simulink model "FLIGHT_hexacopter"  (R2024a)
settings: Solver=FixedStepDiscrete  StartTime=0.0  StopTime=inf  FixedStep=SampleTime_SAS  RelTol=1e-3  EnableMultiTasking=on
InitFcn:
  | Init_FLIGHT_Hexacopter
values from neighbouring files (symbols this model uses):
  d2r = pi/180    (= 0.0174532925199)    [Init_FLIGHT_Hexacopter.m]
  Kdpr = 0.004    [Init_FLIGHT_Hexacopter_fromNCMS.m]
  Kdrr = 0.004    [Init_FLIGHT_Hexacopter_fromNCMS.m]
  Kdvz = 0.0254    [Init_FLIGHT_Hexacopter_fromNCMS.m]
  Kdyr = 0.0298    [Init_FLIGHT_Hexacopter_fromNCMS.m]
  Kipr = 0.0    (= 0)    [Init_FLIGHT_Hexacopter_fromNCMS.m]
  Kirr = 0.0    (= 0)    [Init_FLIGHT_Hexacopter_fromNCMS.m]
  Kivz = 0.6304    [Init_FLIGHT_Hexacopter_fromNCMS.m]
  Kiyr = 0.0    (= 0)    [Init_FLIGHT_Hexacopter_fromNCMS.m]
  Kpp = 3.3894    [Init_FLIGHT_Hexacopter_fromNCMS.m]
  Kppr = 0.1    [Init_FLIGHT_Hexacopter_fromNCMS.m]
  Kpr = 3.3894    [Init_FLIGHT_Hexacopter_fromNCMS.m]
  Kprr = 0.1    [Init_FLIGHT_Hexacopter_fromNCMS.m]
  Kpvz = 0.3191    [Init_FLIGHT_Hexacopter_fromNCMS.m]
  Kpyr = 0.3744    [Init_FLIGHT_Hexacopter_fromNCMS.m]
  MAX_CONTROL_ANGLE_PITCH = 30*pi/180    (= 0.523598775598)    [Init_FLIGHT_Hexacopter.m]    (also in Init_FLIGHT_Hexacopter_fromNCMS.m = 0.349065850399)
  MAX_CONTROL_ANGLE_RATE_PITCH = 360*pi/180    (= 6.28318530718)    [Init_FLIGHT_Hexacopter.m]    (also in Init_FLIGHT_Hexacopter_fromNCMS.m)
  MAX_CONTROL_ANGLE_RATE_ROLL = 360*pi/180    (= 6.28318530718)    [Init_FLIGHT_Hexacopter.m]    (also in Init_FLIGHT_Hexacopter_fromNCMS.m)
  MAX_CONTROL_ANGLE_RATE_Y = 120*pi/180    (= 2.09439510239)    [Init_FLIGHT_Hexacopter.m]    (also in Init_FLIGHT_Hexacopter_fromNCMS.m)
  MAX_CONTROL_ANGLE_ROLL = 30*pi/180    (= 0.523598775598)    [Init_FLIGHT_Hexacopter.m]    (also in Init_FLIGHT_Hexacopter_fromNCMS.m = 0.349065850399)
  MAX_CONTROL_VELOCITY_XY = 1.5    [Init_FLIGHT_Hexacopter.m]    (also in Init_FLIGHT_Hexacopter_fromNCMS.m)
  MAX_CONTROL_VELOCITY_Z = 1    [Init_FLIGHT_Hexacopter.m]    (also in Init_FLIGHT_Hexacopter_fromNCMS.m)
  Npr = 50    [Init_FLIGHT_Hexacopter_fromNCMS.m]
  Nrr = 50    [Init_FLIGHT_Hexacopter_fromNCMS.m]
  Nvz = Npr    (= 50)    [Init_FLIGHT_Hexacopter_fromNCMS.m]
  Nyr = 50    [Init_FLIGHT_Hexacopter_fromNCMS.m]
  SampleTime = 1/200    (= 0.005)    [Init_FLIGHT_Hexacopter.m]    (also in Init_FLIGHT_Hexacopter_fromNCMS.m = 0.01)
  SampleTime_SAS = 1/1000    (= 0.001)    [Init_FLIGHT_Hexacopter.m]
undefined symbols (not defined in the file or in its folder): arguments, event_sequence, id, log_levels, MPC_Z_D, MPC_Z_I, MPC_Z_P, noutputs, output, pitch, pitch_body, q_d, roll, roll_body, thrust_body, timestamp, vx, vy, vz, x, y, yaw, yaw_sp_move_rate, z
libraries: px4lib x35, px4uORBlib x12, px4Utilslib x11, slpidlib x10, simulink x3, simulink_extras x2, px4Sensorslib x2, sharedtransform x1
(part 2 of 3)

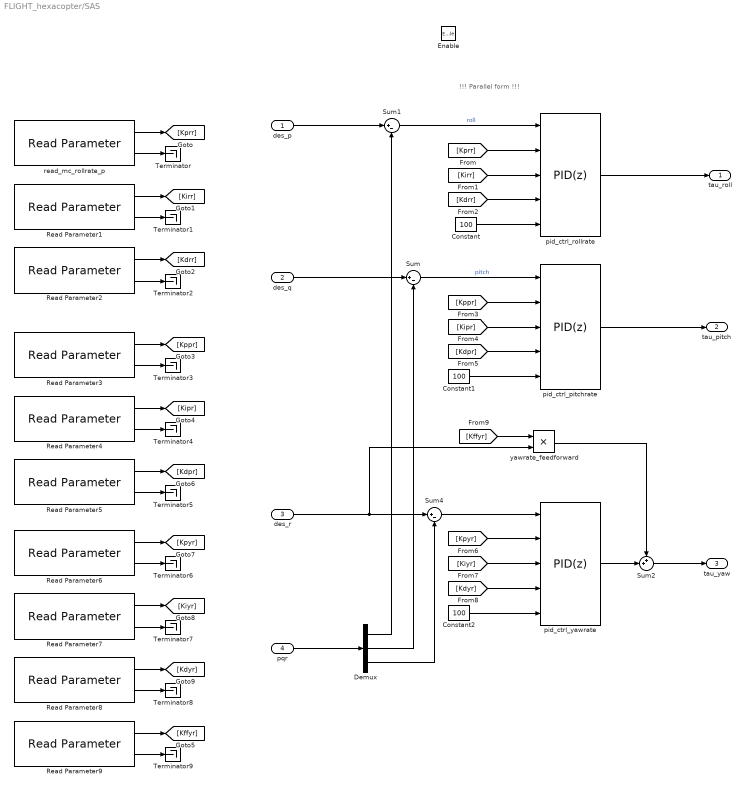
== system FLIGHT_hexacopter/SAS ==
  note: !!! Parallel form !!!
  des_p : Inport
  des_q : Inport  Port=2
  des_r : Inport  Port=3
  pqr : Inport  Port=4
  Enable : EnablePort
  Constant : Constant  Value=100  OutDataTypeStr=single  SampleTime=SampleTime_SAS
  Constant1 : Constant  Value=100  OutDataTypeStr=single  SampleTime=SampleTime_SAS
  Constant2 : Constant  Value=100  OutDataTypeStr=single  SampleTime=SampleTime_SAS
  Demux : Demux  Outputs=3
  Read Parameter1 : px4lib/Read Parameter  ParameterName=MC_ROLLRATE_I  DataType=FLOAT  SampleTime=SampleTime_SAS
      settings: SourceProductName=UAV Toolbox Support Package for PX4 Autopilots
  Read Parameter2 : px4lib/Read Parameter  ParameterName=MC_ROLLRATE_D  DataType=FLOAT  SampleTime=SampleTime_SAS
      settings: SourceProductName=UAV Toolbox Support Package for PX4 Autopilots
  Read Parameter3 : px4lib/Read Parameter  ParameterName=MC_PITCHRATE_P  DataType=FLOAT  SampleTime=SampleTime_SAS
      settings: SourceProductName=UAV Toolbox Support Package for PX4 Autopilots
  Read Parameter4 : px4lib/Read Parameter  ParameterName=MC_PITCHRATE_I  DataType=FLOAT  SampleTime=SampleTime_SAS
      settings: SourceProductName=UAV Toolbox Support Package for PX4 Autopilots
  Read Parameter5 : px4lib/Read Parameter  ParameterName=MC_PITCHRATE_D  DataType=FLOAT  SampleTime=SampleTime_SAS
      settings: SourceProductName=UAV Toolbox Support Package for PX4 Autopilots
  Read Parameter6 : px4lib/Read Parameter  ParameterName=MC_YAWRATE_P  DataType=FLOAT  SampleTime=SampleTime_SAS
      settings: SourceProductName=UAV Toolbox Support Package for PX4 Autopilots
  Read Parameter7 : px4lib/Read Parameter  ParameterName=MC_YAWRATE_I  DataType=FLOAT  SampleTime=SampleTime_SAS
      settings: SourceProductName=UAV Toolbox Support Package for PX4 Autopilots
  Read Parameter8 : px4lib/Read Parameter  ParameterName=MC_YAWRATE_D  DataType=FLOAT  SampleTime=SampleTime_SAS
      settings: SourceProductName=UAV Toolbox Support Package for PX4 Autopilots
  Read Parameter9 : px4lib/Read Parameter  ParameterName=MC_YAWRATE_FF  DataType=FLOAT  SampleTime=SampleTime_SAS
      settings: SourceProductName=UAV Toolbox Support Package for PX4 Autopilots
  Sum : Sum  Inputs=|+-
  Sum1 : Sum  Inputs=|+-
  Sum2 : Sum  Inputs=++|
  Sum4 : Sum  Inputs=|+-
  Terminator{,1..9} (10 alike) : Terminator
  pid_ctrl_pitchrate : slpidlib/PID Controller  Controller=PID  Form=Parallel  TimeDomain=Discrete-time  UseExternalTs=off  SampleTime=SampleTime_SAS  IntegratorMethod=Forward Euler  FilterMethod=Forward Euler  ControllerParametersSource=external  P=Kppr  I=Kipr  UseKiTs=off  D=Kdpr  UseExternalDerivativeSource=off  N=Npr  UseFilter=on  TunerSelectOption=Transfer Function Based (PID Tuner App)  InitialConditionSource=internal  InitialConditionForIntegrator=0  InitialConditionForFilter=0  DifferentiatorICPrevScaledInput=0  ExternalReset=none  TrackingMode=off  Kt=1  LimitOutput=off  SatLimitsSource=internal  UpperSaturationLimit=0.2  LowerSaturationLimit=-0.2  LinearizeAsGain=on  AntiWindupMode=clamping  Kb=1  LimitIntegrator=off  UpperIntegratorSaturationLimit=inf  LowerIntegratorSaturationLimit=-inf  POutMin=[]  POutMax=[]  IOutMin=[]  IOutMax=[]  DOutMin=[]  DOutMax=[]  NOutMin=[]  NOutMax=[]  SumOutMin=[]  SumOutMax=[]  SaturationOutDataTypeStr=single  SaturationOutMin=[]  SaturationOutMax=[]  PParamMin=[]  PParamMax=[]  IParamMin=[]  IParamMax=[]  DParamMin=[]  DParamMax=[]  NParamMin=[]  NParamMax=[]  KbParamMin=[]  KbParamMax=[]  KtParamMin=[]  KtParamMax=[]  KbOutMin=[]  KbOutMax=[]  KtOutMin=[]  KtOutMax=[]  IntegratorOutMin=[]  IntegratorOutMax=[]  FilterOutMin=[]  FilterOutMax=[]  SumI1OutMin=[]  SumI1OutMax=[]  SumI2OutMin=[]  SumI2OutMax=[]  SumI3OutMin=[]  SumI3OutMax=[]  SumI4OutMin=[]  SumI4OutMax=[]  SumDOutMin=[]  SumDOutMax=[]  DifferentiatorOutMin=[]  DifferentiatorOutMax=[]  FilterDiffOutCoefMin=[]  FilterDiffOutCoefMax=[]  ReciprocalOutMin=[]  ReciprocalOutMax=[]  SumDenOutMin=[]  SumDenOutMax=[]  SumNumOutMin=[]  SumNumOutMax=[]  DivideOutMin=[]  DivideOutMax=[]  UdiffTsProdOutMin=[]  UdiffTsProdOutMax=[]  NTsProdOutMin=[]  NTsProdOutMax=[]  UintegralTsProdOutMin=[]  UintegralTsProdOutMax=[]  UngainTsProdOutMin=[]  UngainTsProdOutMax=[]  ClampingZeroOutDataTypeStr=Inherit: Inherit via back propagation  ClampingZeroOutMin=[]  ClampingZeroOutMax=[]  FilterDenConstantOutDataTypeStr=Inherit: Inherit via back propagation  FilterDenConstantOutMin=[]  FilterDenConstantOutMax=[]  PCopyOutDataTypeStr=Inherit: Inherit via back propagation  PCopyOutMin=[]  PCopyOutMax=[]  NCopyOutDataTypeStr=Inherit: Inherit via back propagation  NCopyOutMin=[]  NCopyOutMax=[]  IntegratorContinuousStateAttributes=''  IntegratorStateMustResolveToSignalObject=off  IntegratorRTWStateStorageClass=Auto  FilterContinuousStateAttributes=''  FilterStateMustResolveToSignalObject=off  FilterRTWStateStorageClass=Auto  ParallelPVariant=ExternalParameters  IdealPVariant=Disabled  IVariant=ExternalParameters  DVariant=ExternalParameters  IntegratorVariant=Discrete  SatVariant=Disabled  AWVariant=Passthrough  PCopyVariant=Disabled  TRVariant=Disabled  FdbkBlocksVariant=Forward  IdealPFdbkVariant=Disabled  SatFdbkVariant=Disabled  DerivativeFilterVariant=ForwardEulerFilter  NVariant=ExternalParameters  NCopyVariant=Disabled  FilterICVariant=InternalICsFilter  IntegratorICVariant=InternalICs  ExternalResetVariant=Disabled  TRSumVariant=Passthrough  SumFdbkVariant=Disabled  SumVariant=Sum_PID  TsampFilterVariant=InternalTs  TsampNgainVariant=Passthrough  TsampIntegralVariant=Disabled_SignalSpec  ExternalSaturationOutDataTypeStr=single  DerivativeSourceVariant=ErrorSignal
  pid_ctrl_rollrate : slpidlib/PID Controller  Controller=PID  Form=Parallel  TimeDomain=Discrete-time  UseExternalTs=off  SampleTime=SampleTime_SAS  IntegratorMethod=Forward Euler  FilterMethod=Forward Euler  ControllerParametersSource=external  P=Kprr  I=Kirr  UseKiTs=off  D=Kdrr  UseExternalDerivativeSource=off  N=Nrr  UseFilter=on  TunerSelectOption=Transfer Function Based (PID Tuner App)  InitialConditionSource=internal  InitialConditionForIntegrator=0  InitialConditionForFilter=0  DifferentiatorICPrevScaledInput=0  ExternalReset=none  TrackingMode=off  Kt=1  LimitOutput=off  SatLimitsSource=internal  UpperSaturationLimit=0.2  LowerSaturationLimit=-0.2  LinearizeAsGain=on  AntiWindupMode=clamping  Kb=1  LimitIntegrator=off  UpperIntegratorSaturationLimit=inf  LowerIntegratorSaturationLimit=-inf  POutMin=[]  POutMax=[]  IOutMin=[]  IOutMax=[]  DOutMin=[]  DOutMax=[]  NOutMin=[]  NOutMax=[]  SumOutMin=[]  SumOutMax=[]  SaturationOutDataTypeStr=single  SaturationOutMin=[]  SaturationOutMax=[]  PParamMin=[]  PParamMax=[]  IParamMin=[]  IParamMax=[]  DParamMin=[]  DParamMax=[]  NParamMin=[]  NParamMax=[]  KbParamMin=[]  KbParamMax=[]  KtParamMin=[]  KtParamMax=[]  KbOutMin=[]  KbOutMax=[]  KtOutMin=[]  KtOutMax=[]  IntegratorOutMin=[]  IntegratorOutMax=[]  FilterOutMin=[]  FilterOutMax=[]  SumI1OutMin=[]  SumI1OutMax=[]  SumI2OutMin=[]  SumI2OutMax=[]  SumI3OutMin=[]  SumI3OutMax=[]  SumI4OutMin=[]  SumI4OutMax=[]  SumDOutMin=[]  SumDOutMax=[]  DifferentiatorOutMin=[]  DifferentiatorOutMax=[]  FilterDiffOutCoefMin=[]  FilterDiffOutCoefMax=[]  ReciprocalOutMin=[]  ReciprocalOutMax=[]  SumDenOutMin=[]  SumDenOutMax=[]  SumNumOutMin=[]  SumNumOutMax=[]  DivideOutMin=[]  DivideOutMax=[]  UdiffTsProdOutMin=[]  UdiffTsProdOutMax=[]  NTsProdOutMin=[]  NTsProdOutMax=[]  UintegralTsProdOutMin=[]  UintegralTsProdOutMax=[]  UngainTsProdOutMin=[]  UngainTsProdOutMax=[]  ClampingZeroOutDataTypeStr=Inherit: Inherit via back propagation  ClampingZeroOutMin=[]  ClampingZeroOutMax=[]  FilterDenConstantOutDataTypeStr=Inherit: Inherit via back propagation  FilterDenConstantOutMin=[]  FilterDenConstantOutMax=[]  PCopyOutDataTypeStr=Inherit: Inherit via back propagation  PCopyOutMin=[]  PCopyOutMax=[]  NCopyOutDataTypeStr=Inherit: Inherit via back propagation  NCopyOutMin=[]  NCopyOutMax=[]  IntegratorContinuousStateAttributes=''  IntegratorStateMustResolveToSignalObject=off  IntegratorRTWStateStorageClass=Auto  FilterContinuousStateAttributes=''  FilterStateMustResolveToSignalObject=off  FilterRTWStateStorageClass=Auto  ParallelPVariant=ExternalParameters  IdealPVariant=Disabled  IVariant=ExternalParameters  DVariant=ExternalParameters  IntegratorVariant=Discrete  SatVariant=Disabled  AWVariant=Passthrough  PCopyVariant=Disabled  TRVariant=Disabled  FdbkBlocksVariant=Forward  IdealPFdbkVariant=Disabled  SatFdbkVariant=Disabled  DerivativeFilterVariant=ForwardEulerFilter  NVariant=ExternalParameters  NCopyVariant=Disabled  FilterICVariant=InternalICsFilter  IntegratorICVariant=InternalICs  ExternalResetVariant=Disabled  TRSumVariant=Passthrough  SumFdbkVariant=Disabled  SumVariant=Sum_PID  TsampFilterVariant=InternalTs  TsampNgainVariant=Passthrough  TsampIntegralVariant=Disabled_SignalSpec  ExternalSaturationOutDataTypeStr=single  DerivativeSourceVariant=ErrorSignal
  pid_ctrl_yawrate : slpidlib/PID Controller  Controller=PID  Form=Parallel  TimeDomain=Discrete-time  UseExternalTs=off  SampleTime=SampleTime_SAS  IntegratorMethod=Forward Euler  FilterMethod=Forward Euler  ControllerParametersSource=external  P=Kpyr  I=Kiyr  UseKiTs=off  D=Kdyr  UseExternalDerivativeSource=off  N=Nyr  UseFilter=on  TunerSelectOption=Transfer Function Based (PID Tuner App)  InitialConditionSource=internal  InitialConditionForIntegrator=0  InitialConditionForFilter=0  DifferentiatorICPrevScaledInput=0  ExternalReset=none  TrackingMode=off  Kt=1  LimitOutput=off  SatLimitsSource=internal  UpperSaturationLimit=0.4  LowerSaturationLimit=-0.4  LinearizeAsGain=on  AntiWindupMode=clamping  Kb=1  LimitIntegrator=off  UpperIntegratorSaturationLimit=inf  LowerIntegratorSaturationLimit=-inf  PGainOutDataTypeStr=single  PProdOutDataTypeStr=single  POutMin=[]  POutMax=[]  IGainOutDataTypeStr=single  IProdOutDataTypeStr=single  IOutMin=[]  IOutMax=[]  DGainOutDataTypeStr=single  DProdOutDataTypeStr=single  DOutMin=[]  DOutMax=[]  NGainOutDataTypeStr=single  NProdOutDataTypeStr=single  NOutMin=[]  NOutMax=[]  SumOutDataTypeStr=single  SumOutMin=[]  SumOutMax=[]  SaturationOutMin=[]  SaturationOutMax=[]  PParamMin=[]  PParamMax=[]  IParamMin=[]  IParamMax=[]  DParamMin=[]  DParamMax=[]  NParamMin=[]  NParamMax=[]  KbParamMin=[]  KbParamMax=[]  KtParamMin=[]  KtParamMax=[]  KbOutMin=[]  KbOutMax=[]  KtOutMin=[]  KtOutMax=[]  IntegratorOutMin=[]  IntegratorOutMax=[]  FilterOutMin=[]  FilterOutMax=[]  SumI1OutMin=[]  SumI1OutMax=[]  SumI2OutMin=[]  SumI2OutMax=[]  SumI3OutMin=[]  SumI3OutMax=[]  SumI4OutMin=[]  SumI4OutMax=[]  SumDOutMin=[]  SumDOutMax=[]  DifferentiatorOutMin=[]  DifferentiatorOutMax=[]  FilterDiffOutCoefMin=[]  FilterDiffOutCoefMax=[]  ReciprocalOutMin=[]  ReciprocalOutMax=[]  SumDenOutMin=[]  SumDenOutMax=[]  SumNumOutMin=[]  SumNumOutMax=[]  DivideOutMin=[]  DivideOutMax=[]  UdiffTsProdOutMin=[]  UdiffTsProdOutMax=[]  NTsProdOutMin=[]  NTsProdOutMax=[]  UintegralTsProdOutMin=[]  UintegralTsProdOutMax=[]  UngainTsProdOutMin=[]  UngainTsProdOutMax=[]  ClampingZeroOutDataTypeStr=Inherit: Inherit via back propagation  ClampingZeroOutMin=[]  ClampingZeroOutMax=[]  FilterDenConstantOutDataTypeStr=Inherit: Inherit via back propagation  FilterDenConstantOutMin=[]  FilterDenConstantOutMax=[]  PCopyOutDataTypeStr=Inherit: Inherit via back propagation  PCopyOutMin=[]  PCopyOutMax=[]  NCopyOutDataTypeStr=Inherit: Inherit via back propagation  NCopyOutMin=[]  NCopyOutMax=[]  IntegratorContinuousStateAttributes=''  IntegratorStateMustResolveToSignalObject=off  IntegratorRTWStateStorageClass=Auto  FilterContinuousStateAttributes=''  FilterStateMustResolveToSignalObject=off  FilterRTWStateStorageClass=Auto  ParallelPVariant=ExternalParameters  IdealPVariant=Disabled  IVariant=ExternalParameters  DVariant=ExternalParameters  IntegratorVariant=Discrete  SatVariant=Disabled  AWVariant=Passthrough  PCopyVariant=Disabled  TRVariant=Disabled  FdbkBlocksVariant=Forward  IdealPFdbkVariant=Disabled  SatFdbkVariant=Disabled  DerivativeFilterVariant=ForwardEulerFilter  NVariant=ExternalParameters  NCopyVariant=Disabled  FilterICVariant=InternalICsFilter  IntegratorICVariant=InternalICs  ExternalResetVariant=Disabled  TRSumVariant=Passthrough  SumFdbkVariant=Disabled  SumVariant=Sum_PID  TsampFilterVariant=InternalTs  TsampNgainVariant=Passthrough  TsampIntegralVariant=Disabled_SignalSpec  ExternalSaturationOutDataTypeStr=Inherit: Same as second input  DerivativeSourceVariant=ErrorSignal
  read_mc_rollrate_p : px4lib/Read Parameter  ParameterName=MC_ROLLRATE_P  DataType=FLOAT  SampleTime=SampleTime_SAS
      settings: SourceProductName=UAV Toolbox Support Package for PX4 Autopilots
  yawrate_feedforward : Product
  tau_roll : Outport
  tau_pitch : Outport  Port=2
  tau_yaw : Outport  Port=3
  wires:
  pid_ctrl_rollrate/1 -> tau_roll/1
  pid_ctrl_pitchrate/1 -> tau_pitch/1
  des_r/1 -> yawrate_feedforward/2, Sum4/1
  Sum4/1 -> pid_ctrl_yawrate/1
  Demux/3 -> Sum4/2
  Sum/1 -> pid_ctrl_pitchrate/1  "pitch"
  Demux/2 -> Sum/2
  Demux/1 -> Sum1/2
  pqr/1 -> Demux/1
  Sum1/1 -> pid_ctrl_rollrate/1  "roll"
  des_p/1 -> Sum1/1
  des_q/1 -> Sum/1
  read_mc_rollrate_p/1 -> [Kprr]
  read_mc_rollrate_p/2 -> Terminator/1
  Read Parameter1/1 -> [Kirr]
  Read Parameter1/2 -> Terminator1/1
  Read Parameter2/1 -> [Kdrr]
  Read Parameter2/2 -> Terminator2/1
  [Kprr] -> pid_ctrl_rollrate/2
  [Kirr] -> pid_ctrl_rollrate/3
  [Kdrr] -> pid_ctrl_rollrate/4
  Constant/1 -> pid_ctrl_rollrate/5
  Read Parameter3/1 -> [Kppr]
  Read Parameter3/2 -> Terminator3/1
  Read Parameter4/1 -> [Kipr]
  Read Parameter4/2 -> Terminator4/1
  Read Parameter5/1 -> [Kdpr]
  Read Parameter5/2 -> Terminator5/1
  [Kppr] -> pid_ctrl_pitchrate/2
  [Kipr] -> pid_ctrl_pitchrate/3
  [Kdpr] -> pid_ctrl_pitchrate/4
  Constant1/1 -> pid_ctrl_pitchrate/5
  Read Parameter6/1 -> [Kpyr]
  Read Parameter6/2 -> Terminator6/1
  Read Parameter7/1 -> [Kiyr]
  Read Parameter7/2 -> Terminator7/1
  Read Parameter8/1 -> [Kdyr]
  Read Parameter8/2 -> Terminator8/1
  [Kpyr] -> pid_ctrl_yawrate/2
  [Kiyr] -> pid_ctrl_yawrate/3
  [Kdyr] -> pid_ctrl_yawrate/4
  Constant2/1 -> pid_ctrl_yawrate/5
  Read Parameter9/1 -> [Kffyr]
  Read Parameter9/2 -> Terminator9/1
  [Kffyr] -> yawrate_feedforward/1
  pid_ctrl_yawrate/1 -> Sum2/2
  Sum2/1 -> tau_yaw/1
  yawrate_feedforward/1 -> Sum2/1

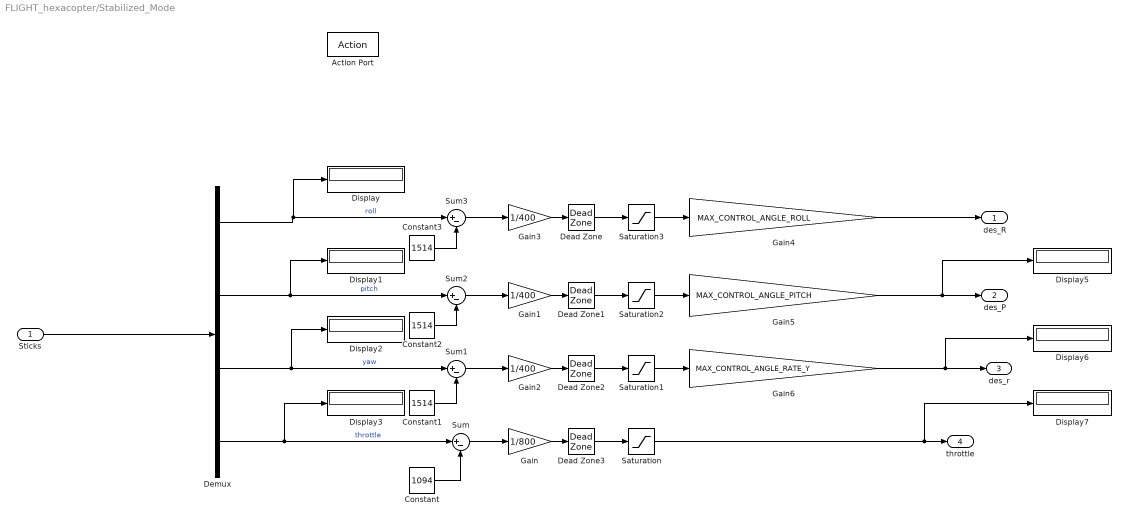
== system FLIGHT_hexacopter/Stabilized_Mode ==
  Sticks : Inport
  Action Port : ActionPort  ActionPortLabel=else
  Constant : Constant  Value=1094
  Constant1 : Constant  Value=1514  OutDataTypeStr=single
  Constant2 : Constant  Value=1514  OutDataTypeStr=single
  Constant3 : Constant  Value=1514  OutDataTypeStr=single
  Dead Zone : DeadZone  LowerValue=-0.005  UpperValue=0.005
  Dead Zone1 : DeadZone  LowerValue=-0.005  UpperValue=0.005
  Dead Zone2 : DeadZone  LowerValue=-0.005  UpperValue=0.005
  Dead Zone3 : DeadZone  LowerValue=-0.05  UpperValue=0.05
  Demux : Demux
  Display{,1..3,5..7} (7 alike) : Display
  Gain : Gain  Gain=1/800  OutDataTypeStr=single
  Gain1 : Gain  Gain=1/400  OutDataTypeStr=single
  Gain2 : Gain  Gain=1/400  OutDataTypeStr=single
  Gain3 : Gain  Gain=1/400  OutDataTypeStr=single
  Gain4 : Gain  Gain=MAX_CONTROL_ANGLE_ROLL
  Gain5 : Gain  Gain=MAX_CONTROL_ANGLE_PITCH
  Gain6 : Gain  Gain=MAX_CONTROL_ANGLE_RATE_Y
  Saturation : Saturate  UpperLimit=0.90  LowerLimit=0
  Saturation1 : Saturate  UpperLimit=1  LowerLimit=-1
  Saturation2 : Saturate  UpperLimit=1  LowerLimit=-1
  Saturation3 : Saturate  UpperLimit=1  LowerLimit=-1
  Sum{,1..3} (4 alike) : Sum  Inputs=|+-
  des_R : Outport
  des_P : Outport  Port=2
  des_r : Outport  Port=3
  throttle : Outport  Port=4
  wires:
  Demux/1 -> Display/1, Sum3/1  "roll"
  Gain3/1 -> Dead Zone/1
  Constant1/1 -> Sum1/2
  Gain/1 -> Dead Zone3/1
  Demux/2 -> Display1/1, Sum2/1  "pitch"
  Gain2/1 -> Dead Zone2/1
  Demux/4 -> Display3/1, Sum/1  "throttle"
  Constant3/1 -> Sum3/2
  Sum3/1 -> Gain3/1
  Constant/1 -> Sum/2
  Sum1/1 -> Gain2/1
  Gain1/1 -> Dead Zone1/1
  Constant2/1 -> Sum2/2
  Demux/3 -> Display2/1, Sum1/1  "yaw"
  Sum/1 -> Gain/1
  Sum2/1 -> Gain1/1
  Sticks/1 -> Demux/1
  Saturation3/1 -> Gain4/1
  Saturation2/1 -> Gain5/1
  Saturation1/1 -> Gain6/1
  Gain6/1 -> Display6/1, des_r/1
  Saturation/1 -> Display7/1, throttle/1
  Dead Zone/1 -> Saturation3/1
  Dead Zone1/1 -> Saturation2/1
  Dead Zone2/1 -> Saturation1/1
  Dead Zone3/1 -> Saturation/1
  Gain5/1 -> Display5/1, des_P/1
  Gain4/1 -> des_R/1

== system FLIGHT_hexacopter/actuator_controls ==
  tau_roll : Inport
  tau_pitch : Inport  Port=2
  tau_yaw : Inport  Port=3
  Ground : Ground
  Mux : Mux  Inputs=3
  PX4 ULog : px4Utilslib/PX4 ULog  uORBTopic=ActuatorControlsStatus
      settings: SourceProductName=PX4 Utility Blocks
  wires:
  Mux/1 -> PX4 ULog/1
  tau_roll/1 -> Mux/1
  tau_pitch/1 -> Mux/2
  tau_yaw/1 -> Mux/3
  Ground/1 -> PX4 ULog/2

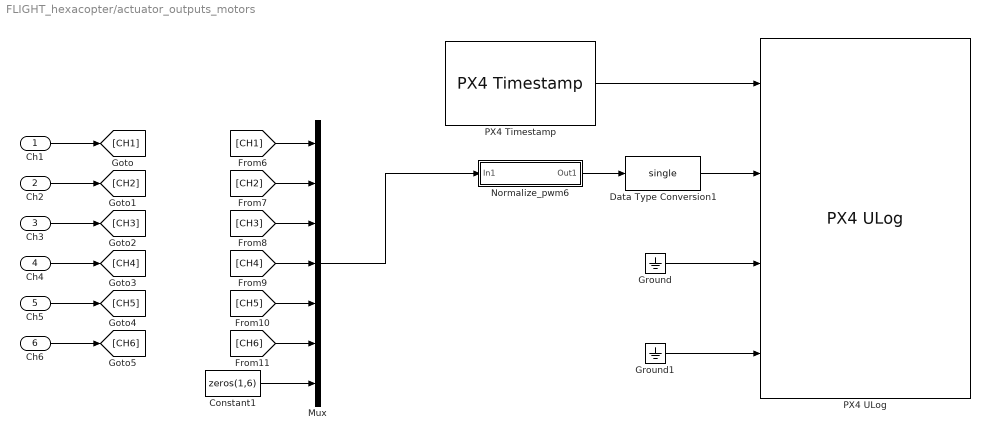
== system FLIGHT_hexacopter/actuator_outputs_motors ==
  Ch1 : Inport
  Ch2 : Inport  Port=2
  Ch3 : Inport  Port=3
  Ch4 : Inport  Port=4
  Ch5 : Inport  Port=5
  Ch6 : Inport  Port=6
  Constant1 : Constant  Value=zeros(1,6)  OutDataTypeStr=single  SampleTime=SampleTime_SAS
  Data Type Conversion1 : DataTypeConversion  OutDataTypeStr=single  SaturateOnIntegerOverflow=off  RndMeth=Floor
  Ground : Ground
  Ground1 : Ground
  Mux : Mux  Inputs=7
  Normalize_pwm6 : Subsystem
  PX4 Timestamp : px4Utilslib/PX4 Timestamp  SampleTime=-1
      settings: SourceProductName=PX4 Utility Blocks
  PX4 ULog : px4Utilslib/PX4 ULog  uORBTopic=ActuatorMotors
      settings: SourceProductName=PX4 Utility Blocks
  wires:
  PX4 Timestamp/1 -> PX4 ULog/1
  Data Type Conversion1/1 -> PX4 ULog/2
  Ground/1 -> PX4 ULog/3
  Ground1/1 -> PX4 ULog/4
  Ch1/1 -> [CH1]
  Ch2/1 -> [CH2]
  Ch3/1 -> [CH3]
  Ch4/1 -> [CH4]
  Ch5/1 -> [CH5]
  Ch6/1 -> [CH6]
  Normalize_pwm6/1(Out1) -> Data Type Conversion1/1
  [CH1] -> Mux/1
  [CH2] -> Mux/2
  [CH3] -> Mux/3
  [CH4] -> Mux/4
  [CH5] -> Mux/5
  [CH6] -> Mux/6
  Mux/1 -> Normalize_pwm6/1(In1)
  Constant1/1 -> Mux/7

== system FLIGHT_hexacopter/sub_vehicle_angular_velocity ==
  Bus Selector2 : BusSelector  OutputSignals=xyz,xyz_derivative
  PX4 uORB Read1 : px4uORBlib/PX4 uORB Read  uORBTopic=VehicleAngularVelocity  selectInstance=vehicle_angular_velocity  SampleTime=SampleTime_SAS  BlockingMode=off  BlockTimeout=1e-3
      settings: SourceProductName=PX4 uORB Read and Write Blocks
  Terminator1 : Terminator
  pqr : Outport
  pqr_dot : Outport  Port=2
  wires:
  PX4 uORB Read1/1 -> Terminator1/1
  Bus Selector2/2 -> pqr_dot/1  "<xyz_derivative>"
  Bus Selector2/1 -> pqr/1  "<xyz>"
  PX4 uORB Read1/2 -> Bus Selector2/1

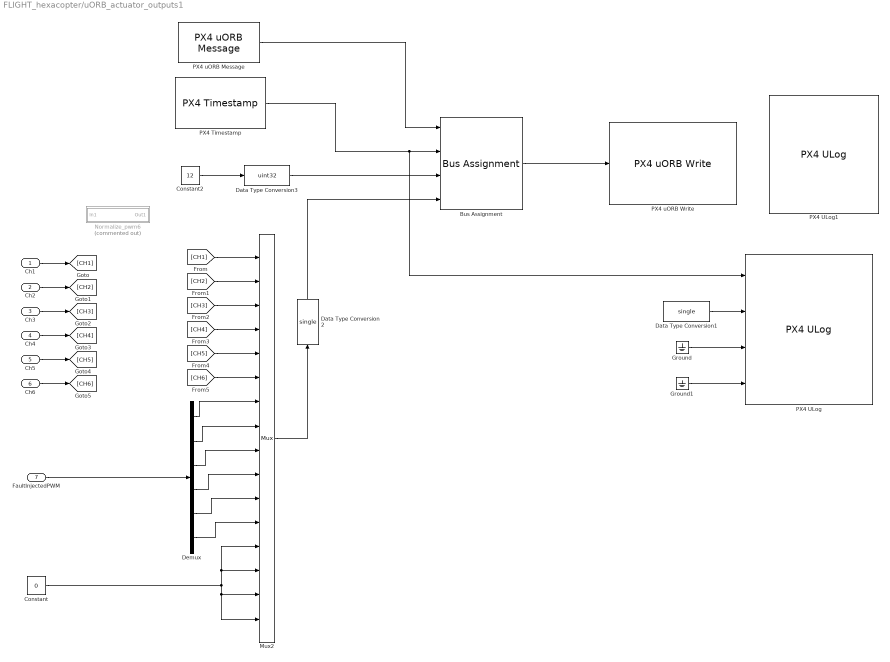
== system FLIGHT_hexacopter/uORB_actuator_outputs1 ==
  Ch1 : Inport
  Ch2 : Inport  Port=2
  Ch3 : Inport  Port=3
  Ch4 : Inport  Port=4
  Ch5 : Inport  Port=5
  Ch6 : Inport  Port=6
  FaultInjectedPWM : Inport  Port=7
  Bus Assignment : BusAssignment  AssignedSignals=timestamp,noutputs,output
  Constant : Constant  Value=0  OutDataTypeStr=single
  Constant2 : Constant  Value=12  OutDataTypeStr=uint32
  Data Type Conversion1 : DataTypeConversion  OutDataTypeStr=single  SaturateOnIntegerOverflow=off  RndMeth=Floor
  Data Type Conversion2 : DataTypeConversion  OutDataTypeStr=single  SaturateOnIntegerOverflow=off  RndMeth=Floor
  Data Type Conversion3 : DataTypeConversion  OutDataTypeStr=uint32  SaturateOnIntegerOverflow=off  RndMeth=Floor
  Demux : Demux  Outputs=6
  Ground : Ground
  Ground1 : Ground
  Mux2 : Mux  Inputs=16
  Normalize_pwm6 : Subsystem  Commented=on
  PX4 Timestamp : px4Utilslib/PX4 Timestamp  SampleTime=-1
      settings: SourceProductName=PX4 Utility Blocks
  PX4 ULog : px4Utilslib/PX4 ULog  uORBTopic=ActuatorMotors
      settings: SourceProductName=PX4 Utility Blocks
  PX4 ULog1 : px4Utilslib/PX4 ULog  uORBTopic=ActuatorOutputs
      settings: SourceProductName=PX4 Utility Blocks
  PX4 uORB Message : px4uORBlib/PX4 uORB Message  uORBTopic=ActuatorOutputs  SampleTime=SampleTime  selectInstance=actuator_outputs
      settings: SourceProductName=PX4 uORB Read and Write Blocks
  PX4 uORB Write : px4uORBlib/PX4 uORB Write  uORBTopic=ActuatorOutputs  selectInstance=actuator_outputs  MessageQueueLen=1
      settings: SourceProductName=PX4 uORB Read and Write Blocks
  wires:
  PX4 uORB Message/1 -> Bus Assignment/1
  Bus Assignment/1 -> PX4 uORB Write/1
  Mux2/1 -> Data Type Conversion2/1
  Constant2/1 -> Data Type Conversion3/1
  Data Type Conversion3/1 -> Bus Assignment/3
  Data Type Conversion2/1 -> Bus Assignment/4
  PX4 Timestamp/1 -> PX4 ULog/1, Bus Assignment/2
  FaultInjectedPWM/1 -> Demux/1
  Demux/1 -> Mux2/7
  Demux/2 -> Mux2/8
  Demux/3 -> Mux2/9
  Demux/4 -> Mux2/10
  Demux/5 -> Mux2/11
  Demux/6 -> Mux2/12
  Constant/1 -> Mux2/16, Mux2/15, Mux2/14, Mux2/13
  Data Type Conversion1/1 -> PX4 ULog/2
  Ground/1 -> PX4 ULog/3
  Ground1/1 -> PX4 ULog/4
  Ch1/1 -> [CH1]
  Ch2/1 -> [CH2]
  Ch3/1 -> [CH3]
  Ch4/1 -> [CH4]
  Ch5/1 -> [CH5]
  Ch6/1 -> [CH6]
  [CH6] -> Mux2/6
  [CH5] -> Mux2/5
  [CH4] -> Mux2/4
  [CH3] -> Mux2/3
  [CH2] -> Mux2/2
  [CH1] -> Mux2/1

== system FLIGHT_hexacopter/vehicle_attitude_setpoint ==
  des_R : Inport
  des_P : Inport  Port=2
  des_Y : Inport  Port=3
  des_thr : Inport  Port=4
  des_r : Inport  Port=5
  Bus Assignment : BusAssignment  AssignedSignals=timestamp,roll_body,pitch_body,yaw_sp_move_rate,thrust_body,q_d
  Constant : Constant  Value=0  OutDataTypeStr=single
  Mux : Mux  Inputs=3
  Mux1 : Mux  Inputs=3
  PX4 Timestamp : px4Utilslib/PX4 Timestamp  SampleTime=-1
      settings: SourceProductName=PX4 Utility Blocks
  PX4 uORB Message : px4uORBlib/PX4 uORB Message  uORBTopic=VehicleAttitudeSetpoint  SampleTime=-1  selectInstance=vehicle_attitude_setpoint
      settings: SourceProductName=PX4 uORB Read and Write Blocks
  PX4 uORB Write : px4uORBlib/PX4 uORB Write  uORBTopic=VehicleAttitudeSetpoint  selectInstance=vehicle_attitude_setpoint  MessageQueueLen=1
      settings: SourceProductName=PX4 uORB Read and Write Blocks
  Rotation Angles to Quaternions : sharedtransform/Rotation Angles to Quaternions  rotationOrder=ZYX  aMode=aMode
  wires:
  PX4 uORB Message/1 -> Bus Assignment/1
  des_thr/1 -> Mux/3
  Constant/1 -> Mux/2, Mux/1
  Mux/1 -> Bus Assignment/6
  Bus Assignment/1 -> PX4 uORB Write/1
  des_Y/1 -> Mux1/1
  des_P/1 -> Bus Assignment/4, Mux1/2
  des_R/1 -> Mux1/3, Bus Assignment/3
  Mux1/1 -> Rotation Angles to Quaternions/1
  Rotation Angles to Quaternions/1 -> Bus Assignment/7
  des_r/1 -> Bus Assignment/5
  PX4 Timestamp/1 -> Bus Assignment/2

== system FLIGHT_hexacopter/vehicle_local_position_setpoint ==
  des_vz : Inport
  des_vxvy : Inport  Port=2
  des_xy : Inport  Port=3
  des_z : Inport  Port=4
  Bus Assignment : BusAssignment  AssignedSignals=timestamp,vx,vy,vz,x,y,z
  Demux : Demux  Outputs=2
  Demux1 : Demux  Outputs=2
  PX4 Timestamp : px4Utilslib/PX4 Timestamp  SampleTime=SampleTime
      settings: SourceProductName=PX4 Utility Blocks
  PX4 uORB Message : px4uORBlib/PX4 uORB Message  uORBTopic=VehicleLocalPositionSetpoint  SampleTime=SampleTime  selectInstance=VehicleLocalPositionSetpoint
      settings: SourceProductName=PX4 uORB Read and Write Blocks
  PX4 uORB Write : px4uORBlib/PX4 uORB Write  uORBTopic=VehicleLocalPositionSetpoint  selectInstance=VehicleLocalPositionSetpoint  MessageQueueLen=1
      settings: SourceProductName=PX4 uORB Read and Write Blocks
  wires:
  PX4 uORB Message/1 -> Bus Assignment/1
  Bus Assignment/1 -> PX4 uORB Write/1
  PX4 Timestamp/1 -> Bus Assignment/2
  des_vz/1 -> Bus Assignment/5
  des_vxvy/1 -> Demux/1
  Demux/1 -> Bus Assignment/3
  Demux/2 -> Bus Assignment/4
  des_xy/1 -> Demux1/1
  Demux1/1 -> Bus Assignment/6
  Demux1/2 -> Bus Assignment/7
  des_z/1 -> Bus Assignment/8

== system FLIGHT_hexacopter/vehicle_rate_setpoint ==
  des_p : Inport
  des_q : Inport  Port=2
  des_r : Inport  Port=3
  des_thr : Inport  Port=4
  Bus Assignment : BusAssignment  AssignedSignals=timestamp,roll,pitch,yaw,thrust_body
  Constant : Constant  Value=0  OutDataTypeStr=single
  Mux : Mux  Inputs=3
  PX4 Timestamp : px4Utilslib/PX4 Timestamp  SampleTime=-1
      settings: SourceProductName=PX4 Utility Blocks
  PX4 uORB Message : px4uORBlib/PX4 uORB Message  uORBTopic=VehicleRatesSetpoint  SampleTime=-1  selectInstance=VehicleRatesSetpoint
      settings: SourceProductName=PX4 uORB Read and Write Blocks
  PX4 uORB Write : px4uORBlib/PX4 uORB Write  uORBTopic=VehicleRatesSetpoint  selectInstance=VehicleRatesSetpoint  MessageQueueLen=1
      settings: SourceProductName=PX4 uORB Read and Write Blocks
  wires:
  PX4 uORB Message/1 -> Bus Assignment/1
  des_thr/1 -> Mux/3
  des_p/1 -> Bus Assignment/3
  des_q/1 -> Bus Assignment/4
  des_r/1 -> Bus Assignment/5
  Constant/1 -> Mux/2, Mux/1
  Mux/1 -> Bus Assignment/6
  Bus Assignment/1 -> PX4 uORB Write/1
  PX4 Timestamp/1 -> Bus Assignment/2

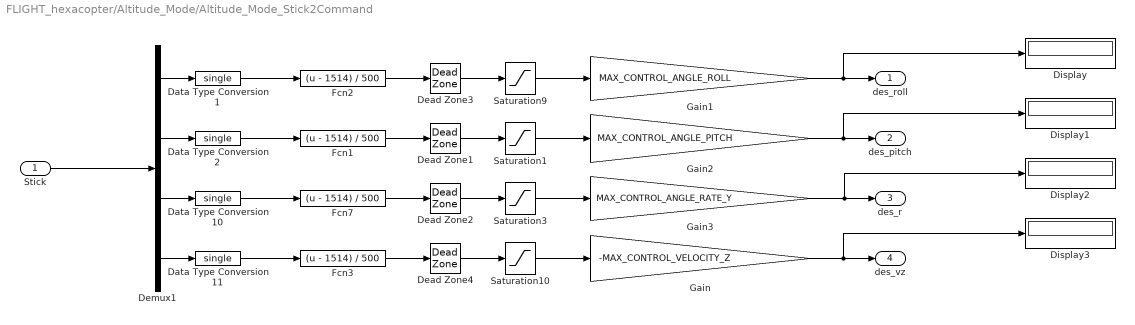
== system FLIGHT_hexacopter/Altitude_Mode/Altitude_Mode_Stick2Command ==
  Stick : Inport
  Data Type Conversion{1..2,10..11} (4 alike) : DataTypeConversion  OutDataTypeStr=single  SaturateOnIntegerOverflow=off  RndMeth=Floor
  Dead Zone1 : DeadZone  LowerValue=-0.001  UpperValue=0.001
  Dead Zone2 : DeadZone  LowerValue=-0.005  UpperValue=0.005
  Dead Zone3 : DeadZone  LowerValue=-0.003  UpperValue=0.003
  Dead Zone4 : DeadZone  LowerValue=-0.03  UpperValue=0.03
  Demux1 : Demux
  Display{,1..3} (4 alike) : Display
  Fcn{1..3,7} (4 alike) : Fcn  Expr=(u - 1514) / 500
  Gain : Gain  Gain=-MAX_CONTROL_VELOCITY_Z
  Gain1 : Gain  Gain=MAX_CONTROL_ANGLE_ROLL
  Gain2 : Gain  Gain=MAX_CONTROL_ANGLE_PITCH
  Gain3 : Gain  Gain=MAX_CONTROL_ANGLE_RATE_Y
  Saturation{1,3,9..10} (4 alike) : Saturate  UpperLimit=1  LowerLimit=-1
  des_roll : Outport
  des_pitch : Outport  Port=2
  des_r : Outport  Port=3
  des_vz : Outport  Port=4
  wires:
  Fcn3/1 -> Dead Zone4/1
  Saturation10/1 -> Gain/1
  Gain1/1 -> Display/1, des_roll/1
  Fcn1/1 -> Dead Zone1/1
  Data Type Conversion1/1 -> Fcn2/1
  Gain2/1 -> Display1/1, des_pitch/1
  Saturation1/1 -> Gain2/1
  Data Type Conversion11/1 -> Fcn3/1
  Dead Zone4/1 -> Saturation10/1
  Gain3/1 -> Display2/1, des_r/1
  Demux1/1 -> Data Type Conversion1/1
  Dead Zone1/1 -> Saturation1/1
  Saturation9/1 -> Gain1/1
  Saturation3/1 -> Gain3/1
  Demux1/4 -> Data Type Conversion11/1
  Data Type Conversion10/1 -> Fcn7/1
  Fcn2/1 -> Dead Zone3/1
  Stick/1 -> Demux1/1
  Demux1/2 -> Data Type Conversion2/1
  Dead Zone3/1 -> Saturation9/1
  Dead Zone2/1 -> Saturation3/1
  Fcn7/1 -> Dead Zone2/1
  Data Type Conversion2/1 -> Fcn1/1
  Demux1/3 -> Data Type Conversion10/1
  Gain/1 -> Display3/1, des_vz/1

== system FLIGHT_hexacopter/Altitude_Mode/Vz Controller ==
  des_vz : Inport
  vz : Inport  Port=2
  Enable : EnablePort
  Constant : Constant  Value=50  OutDataTypeStr=single
  Gain : Gain  Gain=-1
  PID Controller4 : slpidlib/PID Controller  Controller=PID  Form=Parallel  TimeDomain=Discrete-time  UseExternalTs=off  SampleTime=SampleTime  IntegratorMethod=Forward Euler  FilterMethod=Forward Euler  ControllerParametersSource=external  P=1  I=0  UseKiTs=off  D=0  UseExternalDerivativeSource=off  N=50  UseFilter=on  TunerSelectOption=Transfer Function Based (PID Tuner App)  InitialConditionSource=internal  InitialConditionForIntegrator=0  InitialConditionForFilter=0  DifferentiatorICPrevScaledInput=0  ExternalReset=none  TrackingMode=off  Kt=1  LimitOutput=on  SatLimitsSource=internal  UpperSaturationLimit=1  LowerSaturationLimit=-1  LinearizeAsGain=on  AntiWindupMode=clamping  Kb=1  LimitIntegrator=off  UpperIntegratorSaturationLimit=inf  LowerIntegratorSaturationLimit=-inf  POutMin=[]  POutMax=[]  IOutMin=[]  IOutMax=[]  DOutMin=[]  DOutMax=[]  NOutMin=[]  NOutMax=[]  SumOutMin=[]  SumOutMax=[]  SaturationOutMin=[]  SaturationOutMax=[]  PParamMin=[]  PParamMax=[]  IParamMin=[]  IParamMax=[]  DParamMin=[]  DParamMax=[]  NParamMin=[]  NParamMax=[]  KbParamMin=[]  KbParamMax=[]  KtParamMin=[]  KtParamMax=[]  KbOutMin=[]  KbOutMax=[]  KtOutMin=[]  KtOutMax=[]  IntegratorOutMin=[]  IntegratorOutMax=[]  FilterOutMin=[]  FilterOutMax=[]  SumI1OutMin=[]  SumI1OutMax=[]  SumI2OutMin=[]  SumI2OutMax=[]  SumI3OutMin=[]  SumI3OutMax=[]  SumI4OutMin=[]  SumI4OutMax=[]  SumDOutMin=[]  SumDOutMax=[]  DifferentiatorOutMin=[]  DifferentiatorOutMax=[]  FilterDiffOutCoefMin=[]  FilterDiffOutCoefMax=[]  ReciprocalOutMin=[]  ReciprocalOutMax=[]  SumDenOutMin=[]  SumDenOutMax=[]  SumNumOutMin=[]  SumNumOutMax=[]  DivideOutMin=[]  DivideOutMax=[]  UdiffTsProdOutMin=[]  UdiffTsProdOutMax=[]  NTsProdOutMin=[]  NTsProdOutMax=[]  UintegralTsProdOutMin=[]  UintegralTsProdOutMax=[]  UngainTsProdOutMin=[]  UngainTsProdOutMax=[]  ClampingZeroOutDataTypeStr=Inherit: Inherit via back propagation  ClampingZeroOutMin=[]  ClampingZeroOutMax=[]  FilterDenConstantOutDataTypeStr=Inherit: Inherit via back propagation  FilterDenConstantOutMin=[]  FilterDenConstantOutMax=[]  PCopyOutDataTypeStr=Inherit: Inherit via back propagation  PCopyOutMin=[]  PCopyOutMax=[]  NCopyOutDataTypeStr=Inherit: Inherit via back propagation  NCopyOutMin=[]  NCopyOutMax=[]  IntegratorContinuousStateAttributes=''  IntegratorStateMustResolveToSignalObject=off  IntegratorRTWStateStorageClass=Auto  FilterContinuousStateAttributes=''  FilterStateMustResolveToSignalObject=off  FilterRTWStateStorageClass=Auto  ParallelPVariant=ExternalParameters  IdealPVariant=Disabled  IVariant=ExternalParameters  DVariant=ExternalParameters  IntegratorVariant=Discrete  SatVariant=Enabled  AWVariant=DiscClampingParallel  PCopyVariant=Disabled  TRVariant=Disabled  FdbkBlocksVariant=Forward  IdealPFdbkVariant=Disabled  SatFdbkVariant=Disabled  DerivativeFilterVariant=ForwardEulerFilter  NVariant=ExternalParameters  NCopyVariant=Disabled  FilterICVariant=InternalICsFilter  IntegratorICVariant=InternalICs  ExternalResetVariant=Disabled  TRSumVariant=Passthrough  SumFdbkVariant=Disabled  SumVariant=Sum_PID  TsampFilterVariant=InternalTs  TsampNgainVariant=Passthrough  TsampIntegralVariant=Disabled_SignalSpec  ExternalSaturationOutDataTypeStr=Inherit: Same as second input  DerivativeSourceVariant=ErrorSignal
  Read Parameter : px4lib/Read Parameter  ParameterName=MPC_THR_HOVER  DataType=FLOAT  SampleTime=SampleTime
      settings: SourceProductName=UAV Toolbox Support Package for PX4 Autopilots
  Read Parameter1 : px4lib/Read Parameter  ParameterName=MPC_Z_VEL_P_ACC  DataType=FLOAT  SampleTime=SampleTime
      settings: SourceProductName=UAV Toolbox Support Package for PX4 Autopilots
  Read Parameter2 : px4lib/Read Parameter  ParameterName=MPC_Z_VEL_I_ACC  DataType=FLOAT  SampleTime=SampleTime
      settings: SourceProductName=UAV Toolbox Support Package for PX4 Autopilots
  Read Parameter3 : px4lib/Read Parameter  ParameterName=MPC_Z_VEL_D_ACC  DataType=FLOAT  SampleTime=SampleTime
      settings: SourceProductName=UAV Toolbox Support Package for PX4 Autopilots
  Saturation1 : Saturate  UpperLimit=1  LowerLimit=0  OutDataTypeStr=single
  Sum3 : Sum  Inputs=|+-
  Sum6 : Sum  Inputs=|++  OutDataTypeStr=single
  Terminator{,1..3} (4 alike) : Terminator
  throttle : Outport  OutDataTypeStr=single
  wires:
  vz/1 -> Sum3/2
  des_vz/1 -> Sum3/1
  Sum3/1 -> Gain/1
  Gain/1 -> PID Controller4/1
  PID Controller4/1 -> Sum6/1
  Sum6/1 -> Saturation1/1
  Read Parameter/1 -> Sum6/2
  Read Parameter/2 -> Terminator/1
  Read Parameter1/1 -> [kpz]
  Read Parameter2/1 -> [Kiz]
  Read Parameter3/1 -> [Kdz]
  Read Parameter1/2 -> Terminator1/1
  Read Parameter2/2 -> Terminator2/1
  Read Parameter3/2 -> Terminator3/1
  Saturation1/1 -> throttle/1
  [kpz] -> PID Controller4/2
  [Kiz] -> PID Controller4/3
  [Kdz] -> PID Controller4/4
  Constant/1 -> PID Controller4/5

== system FLIGHT_hexacopter/Fault_Injection/Send Fault Injection to QGC ==
  Inject : Inport
  Bus Assignment : BusAssignment  AssignedSignals=timestamp,id,event_sequence,arguments,log_levels
  PX4 Timestamp : px4Utilslib/PX4 Timestamp  SampleTime=SampleTime
  PX4 uORB Message : px4uORBlib/PX4 uORB Message  uORBTopic=Event  SampleTime=inf  selectInstance=Event
  PX4 uORB Write : px4uORBlib/PX4 uORB Write  uORBTopic=FailsafeFlags  selectInstance=FailsafeFlags  MessageQueueLen=1
  wires:
  PX4 uORB Message/1 -> Bus Assignment/1
  Bus Assignment/1 -> PX4 uORB Write/1
  PX4 Timestamp/1 -> Bus Assignment/2

== system FLIGHT_hexacopter/If Action Subsystem/Altitude Controller ==
  des_z : Inport
  z : Inport  Port=2
  Enable : EnablePort
  PID Controller4 : slpidlib/PID Controller  Controller=P  Form=Parallel  TimeDomain=Discrete-time  UseExternalTs=off  SampleTime=SampleTime  IntegratorMethod=Forward Euler  FilterMethod=Forward Euler  ControllerParametersSource=external  P=Kpvz  I=Kivz  UseKiTs=off  D=Kdvz  UseExternalDerivativeSource=off  N=Nvz  UseFilter=on  TunerSelectOption=Transfer Function Based (PID Tuner App)  InitialConditionSource=internal  InitialConditionForIntegrator=0  InitialConditionForFilter=0  DifferentiatorICPrevScaledInput=0  ExternalReset=none  TrackingMode=off  Kt=1  LimitOutput=on  SatLimitsSource=internal  UpperSaturationLimit=1  LowerSaturationLimit=-1  LinearizeAsGain=on  AntiWindupMode=clamping  Kb=1  LimitIntegrator=off  UpperIntegratorSaturationLimit=inf  LowerIntegratorSaturationLimit=-inf  POutMin=[]  POutMax=[]  IOutMin=[]  IOutMax=[]  DOutMin=[]  DOutMax=[]  NOutMin=[]  NOutMax=[]  SumOutMin=[]  SumOutMax=[]  SaturationOutMin=[]  SaturationOutMax=[]  PParamMin=[]  PParamMax=[]  IParamMin=[]  IParamMax=[]  DParamMin=[]  DParamMax=[]  NParamMin=[]  NParamMax=[]  KbParamMin=[]  KbParamMax=[]  KtParamMin=[]  KtParamMax=[]  KbOutMin=[]  KbOutMax=[]  KtOutMin=[]  KtOutMax=[]  IntegratorOutMin=[]  IntegratorOutMax=[]  FilterOutMin=[]  FilterOutMax=[]  SumI1OutMin=[]  SumI1OutMax=[]  SumI2OutMin=[]  SumI2OutMax=[]  SumI3OutMin=[]  SumI3OutMax=[]  SumI4OutMin=[]  SumI4OutMax=[]  SumDOutMin=[]  SumDOutMax=[]  DifferentiatorOutMin=[]  DifferentiatorOutMax=[]  FilterDiffOutCoefMin=[]  FilterDiffOutCoefMax=[]  ReciprocalOutMin=[]  ReciprocalOutMax=[]  SumDenOutMin=[]  SumDenOutMax=[]  SumNumOutMin=[]  SumNumOutMax=[]  DivideOutMin=[]  DivideOutMax=[]  UdiffTsProdOutMin=[]  UdiffTsProdOutMax=[]  NTsProdOutMin=[]  NTsProdOutMax=[]  UintegralTsProdOutMin=[]  UintegralTsProdOutMax=[]  UngainTsProdOutMin=[]  UngainTsProdOutMax=[]  ClampingZeroOutDataTypeStr=Inherit: Inherit via back propagation  ClampingZeroOutMin=[]  ClampingZeroOutMax=[]  FilterDenConstantOutDataTypeStr=Inherit: Inherit via back propagation  FilterDenConstantOutMin=[]  FilterDenConstantOutMax=[]  PCopyOutDataTypeStr=Inherit: Inherit via back propagation  PCopyOutMin=[]  PCopyOutMax=[]  NCopyOutDataTypeStr=Inherit: Inherit via back propagation  NCopyOutMin=[]  NCopyOutMax=[]  IntegratorContinuousStateAttributes=''  IntegratorStateMustResolveToSignalObject=off  IntegratorRTWStateStorageClass=Auto  FilterContinuousStateAttributes=''  FilterStateMustResolveToSignalObject=off  FilterRTWStateStorageClass=Auto  ParallelPVariant=ExternalParameters  IdealPVariant=Disabled  IVariant=Disabled  DVariant=Disabled  IntegratorVariant=Disabled  SatVariant=Enabled  AWVariant=Disabled  PCopyVariant=Disabled  TRVariant=Disabled  FdbkBlocksVariant=Forward  IdealPFdbkVariant=Disabled  SatFdbkVariant=Disabled  DerivativeFilterVariant=Disabled  NVariant=Disabled  NCopyVariant=Disabled_SignalSpec  FilterICVariant=Disabled  IntegratorICVariant=Disabled  ExternalResetVariant=Disabled  TRSumVariant=Passthrough  SumFdbkVariant=Disabled  SumVariant=Passthrough_P  TsampFilterVariant=InternalTs  TsampNgainVariant=Passthrough  TsampIntegralVariant=Disabled_SignalSpec  ExternalSaturationOutDataTypeStr=Inherit: Same as second input  DerivativeSourceVariant=Disabled
  Read Parameter1 : px4lib/Read Parameter  ParameterName=MPC_Z_P  DataType=FLOAT  SampleTime=SampleTime
      settings: SourceProductName=UAV Toolbox Support Package for PX4 Autopilots
  Sum : Sum  Inputs=|+-
  Terminator1 : Terminator
  des_vz : Outport
  wires:
  Read Parameter1/1 -> [kpz]
  Read Parameter1/2 -> Terminator1/1
  [kpz] -> PID Controller4/2
  PID Controller4/1 -> des_vz/1
  des_z/1 -> Sum/1
  Sum/1 -> PID Controller4/1
  z/1 -> Sum/2

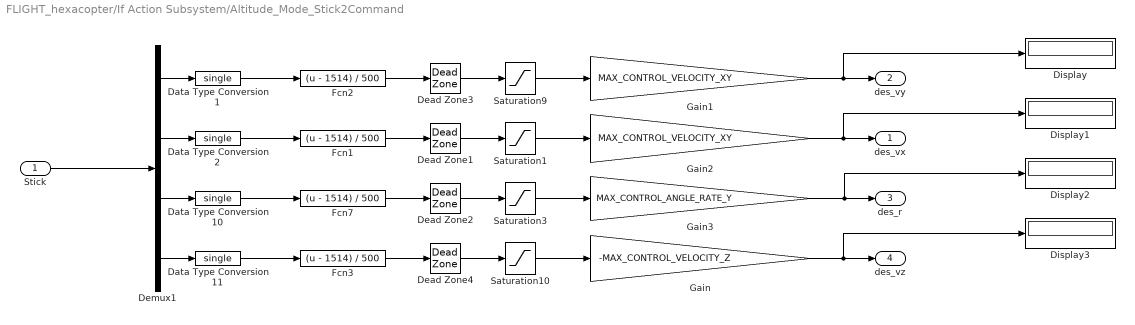
== system FLIGHT_hexacopter/If Action Subsystem/Altitude_Mode_Stick2Command ==
  Stick : Inport
  Data Type Conversion{1..2,10..11} (4 alike) : DataTypeConversion  OutDataTypeStr=single  SaturateOnIntegerOverflow=off  RndMeth=Floor
  Dead Zone{1..4} (4 alike) : DeadZone  LowerValue=-0.1  UpperValue=0.1
  Demux1 : Demux
  Display{,1..3} (4 alike) : Display
  Fcn{1..3,7} (4 alike) : Fcn  Expr=(u - 1514) / 500
  Gain : Gain  Gain=-MAX_CONTROL_VELOCITY_Z
  Gain1 : Gain  Gain=MAX_CONTROL_VELOCITY_XY
  Gain2 : Gain  Gain=MAX_CONTROL_VELOCITY_XY
  Gain3 : Gain  Gain=MAX_CONTROL_ANGLE_RATE_Y
  Saturation{1,3,9..10} (4 alike) : Saturate  UpperLimit=1  LowerLimit=-1
  des_vx : Outport
  des_vy : Outport  Port=2
  des_r : Outport  Port=3
  des_vz : Outport  Port=4
  wires:
  Fcn3/1 -> Dead Zone4/1
  Saturation10/1 -> Gain/1
  Gain1/1 -> Display/1, des_vy/1
  Fcn1/1 -> Dead Zone1/1
  Data Type Conversion1/1 -> Fcn2/1
  Gain2/1 -> Display1/1, des_vx/1
  Saturation1/1 -> Gain2/1
  Data Type Conversion11/1 -> Fcn3/1
  Dead Zone4/1 -> Saturation10/1
  Gain3/1 -> Display2/1, des_r/1
  Demux1/1 -> Data Type Conversion1/1
  Dead Zone1/1 -> Saturation1/1
  Saturation9/1 -> Gain1/1
  Saturation3/1 -> Gain3/1
  Demux1/4 -> Data Type Conversion11/1
  Data Type Conversion10/1 -> Fcn7/1
  Fcn2/1 -> Dead Zone3/1
  Stick/1 -> Demux1/1
  Demux1/2 -> Data Type Conversion2/1
  Dead Zone3/1 -> Saturation9/1
  Dead Zone2/1 -> Saturation3/1
  Fcn7/1 -> Dead Zone2/1
  Data Type Conversion2/1 -> Fcn1/1
  Demux1/3 -> Data Type Conversion10/1
  Gain/1 -> Display3/1, des_vz/1

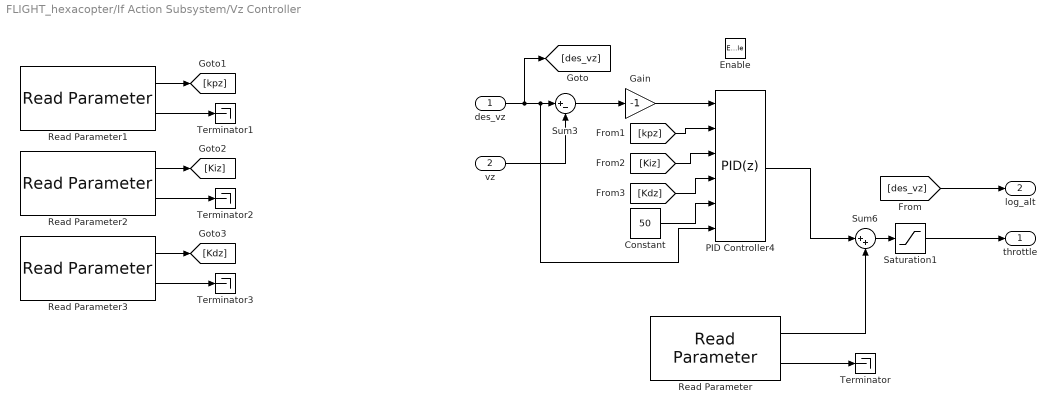
== system FLIGHT_hexacopter/If Action Subsystem/Vz Controller ==
  des_vz : Inport
  vz : Inport  Port=2
  Enable : EnablePort
  Constant : Constant  Value=50  OutDataTypeStr=single
  Gain : Gain  Gain=-1
  PID Controller4 : slpidlib/PID Controller  Controller=PID  Form=Parallel  TimeDomain=Discrete-time  UseExternalTs=off  SampleTime=SampleTime  IntegratorMethod=Forward Euler  FilterMethod=Forward Euler  ControllerParametersSource=external  P=Kpvz  I=Kivz  UseKiTs=off  D=Kdvz  UseExternalDerivativeSource=off  N=Nvz  UseFilter=on  TunerSelectOption=Transfer Function Based (PID Tuner App)  InitialConditionSource=internal  InitialConditionForIntegrator=0  InitialConditionForFilter=0  DifferentiatorICPrevScaledInput=0  ExternalReset=rising  TrackingMode=off  Kt=1  LimitOutput=on  SatLimitsSource=internal  UpperSaturationLimit=1  LowerSaturationLimit=-1  LinearizeAsGain=on  AntiWindupMode=clamping  Kb=1  LimitIntegrator=off  UpperIntegratorSaturationLimit=inf  LowerIntegratorSaturationLimit=-inf  POutMin=[]  POutMax=[]  IOutMin=[]  IOutMax=[]  DOutMin=[]  DOutMax=[]  NOutMin=[]  NOutMax=[]  SumOutMin=[]  SumOutMax=[]  SaturationOutMin=[]  SaturationOutMax=[]  PParamMin=[]  PParamMax=[]  IParamMin=[]  IParamMax=[]  DParamMin=[]  DParamMax=[]  NParamMin=[]  NParamMax=[]  KbParamMin=[]  KbParamMax=[]  KtParamMin=[]  KtParamMax=[]  KbOutMin=[]  KbOutMax=[]  KtOutMin=[]  KtOutMax=[]  IntegratorOutMin=[]  IntegratorOutMax=[]  FilterOutMin=[]  FilterOutMax=[]  SumI1OutMin=[]  SumI1OutMax=[]  SumI2OutMin=[]  SumI2OutMax=[]  SumI3OutMin=[]  SumI3OutMax=[]  SumI4OutMin=[]  SumI4OutMax=[]  SumDOutMin=[]  SumDOutMax=[]  DifferentiatorOutMin=[]  DifferentiatorOutMax=[]  FilterDiffOutCoefMin=[]  FilterDiffOutCoefMax=[]  ReciprocalOutMin=[]  ReciprocalOutMax=[]  SumDenOutMin=[]  SumDenOutMax=[]  SumNumOutMin=[]  SumNumOutMax=[]  DivideOutMin=[]  DivideOutMax=[]  UdiffTsProdOutMin=[]  UdiffTsProdOutMax=[]  NTsProdOutMin=[]  NTsProdOutMax=[]  UintegralTsProdOutMin=[]  UintegralTsProdOutMax=[]  UngainTsProdOutMin=[]  UngainTsProdOutMax=[]  ClampingZeroOutDataTypeStr=Inherit: Inherit via back propagation  ClampingZeroOutMin=[]  ClampingZeroOutMax=[]  FilterDenConstantOutDataTypeStr=Inherit: Inherit via back propagation  FilterDenConstantOutMin=[]  FilterDenConstantOutMax=[]  PCopyOutDataTypeStr=Inherit: Inherit via back propagation  PCopyOutMin=[]  PCopyOutMax=[]  NCopyOutDataTypeStr=Inherit: Inherit via back propagation  NCopyOutMin=[]  NCopyOutMax=[]  IntegratorContinuousStateAttributes=''  IntegratorStateMustResolveToSignalObject=off  IntegratorRTWStateStorageClass=Auto  FilterContinuousStateAttributes=''  FilterStateMustResolveToSignalObject=off  FilterRTWStateStorageClass=Auto  ParallelPVariant=ExternalParameters  IdealPVariant=Disabled  IVariant=ExternalParameters  DVariant=ExternalParameters  IntegratorVariant=Discrete  SatVariant=Enabled  AWVariant=DiscClampingParallel  PCopyVariant=Disabled  TRVariant=Disabled  FdbkBlocksVariant=Forward  IdealPFdbkVariant=Disabled  SatFdbkVariant=Disabled  DerivativeFilterVariant=ForwardEulerFilter  NVariant=ExternalParameters  NCopyVariant=Disabled  FilterICVariant=InternalICsFilter  IntegratorICVariant=InternalICs  ExternalResetVariant=ExternalReset  TRSumVariant=Passthrough  SumFdbkVariant=Disabled  SumVariant=Sum_PID  TsampFilterVariant=InternalTs  TsampNgainVariant=Passthrough  TsampIntegralVariant=Disabled_SignalSpec  ExternalSaturationOutDataTypeStr=Inherit: Same as second input  DerivativeSourceVariant=ErrorSignal
  Read Parameter : px4lib/Read Parameter  ParameterName=MPC_THR_HOVER  DataType=FLOAT  SampleTime=SampleTime
      settings: SourceProductName=UAV Toolbox Support Package for PX4 Autopilots
  Read Parameter1 : px4lib/Read Parameter  ParameterName=MPC_Z_VEL_P_ACC  DataType=FLOAT  SampleTime=SampleTime
      settings: SourceProductName=UAV Toolbox Support Package for PX4 Autopilots
  Read Parameter2 : px4lib/Read Parameter  ParameterName=MPC_Z_VEL_I_ACC  DataType=FLOAT  SampleTime=SampleTime
      settings: SourceProductName=UAV Toolbox Support Package for PX4 Autopilots
  Read Parameter3 : px4lib/Read Parameter  ParameterName=MPC_Z_VEL_D_ACC  DataType=FLOAT  SampleTime=SampleTime
      settings: SourceProductName=UAV Toolbox Support Package for PX4 Autopilots
  Saturation1 : Saturate  UpperLimit=1  LowerLimit=0  OutDataTypeStr=single
  Sum3 : Sum  Inputs=|+-
  Sum6 : Sum  Inputs=|++  OutDataTypeStr=single
  Terminator{,1..3} (4 alike) : Terminator
  throttle : Outport  OutDataTypeStr=single
  log_alt : Outport  Port=2  OutDataTypeStr=single
  wires:
  vz/1 -> Sum3/2
  des_vz/1 -> [des_vz], PID Controller4/6, Sum3/1
  Sum3/1 -> Gain/1
  Gain/1 -> PID Controller4/1
  PID Controller4/1 -> Sum6/1
  Sum6/1 -> Saturation1/1
  Read Parameter/1 -> Sum6/2
  [des_vz] -> log_alt/1
  Read Parameter/2 -> Terminator/1
  Read Parameter1/1 -> [kpz]
  Read Parameter2/1 -> [Kiz]
  Read Parameter3/1 -> [Kdz]
  Read Parameter1/2 -> Terminator1/1
  Read Parameter2/2 -> Terminator2/1
  Read Parameter3/2 -> Terminator3/1
  [kpz] -> PID Controller4/2
  [Kiz] -> PID Controller4/3
  [Kdz] -> PID Controller4/4
  Constant/1 -> PID Controller4/5
  Saturation1/1 -> throttle/1

== system FLIGHT_hexacopter/If Action Subsystem/XY Pos Controller ==
  des_xy : Inport
  xy : Inport  Port=2
  Enable : EnablePort
  PID_Altitude : slpidlib/PID Controller  Controller=P  Form=Parallel  TimeDomain=Discrete-time  UseExternalTs=off  SampleTime=-1  IntegratorMethod=Backward Euler  FilterMethod=Forward Euler  ControllerParametersSource=external  P=MPC_Z_P  I=MPC_Z_I  UseKiTs=off  D=MPC_Z_D  UseExternalDerivativeSource=off  N=10  UseFilter=on  TunerSelectOption=Transfer Function Based (PID Tuner App)  InitialConditionSource=internal  InitialConditionForIntegrator=0  InitialConditionForFilter=0  DifferentiatorICPrevScaledInput=0  ExternalReset=none  TrackingMode=off  Kt=1  LimitOutput=off  SatLimitsSource=internal  UpperSaturationLimit=inf  LowerSaturationLimit=-inf  LinearizeAsGain=off  AntiWindupMode=clamping  Kb=1  LimitIntegrator=off  UpperIntegratorSaturationLimit=inf  LowerIntegratorSaturationLimit=-inf  POutMin=[]  POutMax=[]  IOutMin=[]  IOutMax=[]  DOutMin=[]  DOutMax=[]  NOutMin=[]  NOutMax=[]  SumOutMin=[]  SumOutMax=[]  SaturationOutMin=[]  SaturationOutMax=[]  PParamMin=[]  PParamMax=[]  IParamMin=[]  IParamMax=[]  DParamMin=[]  DParamMax=[]  NParamMin=[]  NParamMax=[]  KbParamMin=[]  KbParamMax=[]  KtParamMin=[]  KtParamMax=[]  KbOutMin=[]  KbOutMax=[]  KtOutMin=[]  KtOutMax=[]  IntegratorOutMin=[]  IntegratorOutMax=[]  FilterOutMin=[]  FilterOutMax=[]  SumI1OutMin=[]  SumI1OutMax=[]  SumI2OutMin=[]  SumI2OutMax=[]  SumI3OutMin=[]  SumI3OutMax=[]  SumI4OutMin=[]  SumI4OutMax=[]  SumDOutMin=[]  SumDOutMax=[]  DifferentiatorOutMin=[]  DifferentiatorOutMax=[]  FilterDiffOutCoefMin=[]  FilterDiffOutCoefMax=[]  ReciprocalOutMin=[]  ReciprocalOutMax=[]  SumDenOutMin=[]  SumDenOutMax=[]  SumNumOutMin=[]  SumNumOutMax=[]  DivideOutMin=[]  DivideOutMax=[]  UdiffTsProdOutMin=[]  UdiffTsProdOutMax=[]  NTsProdOutMin=[]  NTsProdOutMax=[]  UintegralTsProdOutMin=[]  UintegralTsProdOutMax=[]  UngainTsProdOutMin=[]  UngainTsProdOutMax=[]  ClampingZeroOutDataTypeStr=Inherit: Inherit via back propagation  ClampingZeroOutMin=[]  ClampingZeroOutMax=[]  FilterDenConstantOutDataTypeStr=Inherit: Inherit via back propagation  FilterDenConstantOutMin=[]  FilterDenConstantOutMax=[]  PCopyOutDataTypeStr=Inherit: Inherit via back propagation  PCopyOutMin=[]  PCopyOutMax=[]  NCopyOutDataTypeStr=Inherit: Inherit via back propagation  NCopyOutMin=[]  NCopyOutMax=[]  IntegratorContinuousStateAttributes=''  IntegratorStateMustResolveToSignalObject=off  IntegratorRTWStateStorageClass=Auto  FilterContinuousStateAttributes=''  FilterStateMustResolveToSignalObject=off  FilterRTWStateStorageClass=Auto  ParallelPVariant=ExternalParameters  IdealPVariant=Disabled  IVariant=Disabled  DVariant=Disabled  IntegratorVariant=Disabled  SatVariant=Disabled  AWVariant=Disabled  PCopyVariant=Disabled  TRVariant=Disabled  FdbkBlocksVariant=Forward  IdealPFdbkVariant=Disabled  SatFdbkVariant=Disabled  DerivativeFilterVariant=Disabled  NVariant=Disabled  NCopyVariant=Disabled_SignalSpec  FilterICVariant=Disabled  IntegratorICVariant=Disabled  ExternalResetVariant=Disabled  TRSumVariant=Passthrough  SumFdbkVariant=Disabled  SumVariant=Passthrough_P  TsampFilterVariant=InternalTs  TsampNgainVariant=Passthrough  TsampIntegralVariant=Disabled_SignalSpec  ExternalSaturationOutDataTypeStr=Inherit: Same as second input  DerivativeSourceVariant=Disabled
  Read Parameter : px4lib/Read Parameter  ParameterName=MPC_XY_P  DataType=FLOAT  SampleTime=SampleTime
      settings: SourceProductName=UAV Toolbox Support Package for PX4 Autopilots
  Sum : Sum  Inputs=|+-
  Terminator : Terminator
  des_vxvy : Outport
  wires:
  PID_Altitude/1 -> des_vxvy/1  "vz_cmd"
  Read Parameter/1 -> PID_Altitude/2
  des_xy/1 -> Sum/1
  Sum/1 -> PID_Altitude/1
  xy/1 -> Sum/2
  Read Parameter/2 -> Terminator/1
